simulink model "filt_adapt"  (R2020a)
settings: Solver=VariableStepAuto  StartTime=0.0  StopTime=10.0  RelTol=1e-3
values from neighbouring files (symbols this model uses):
  miu = 0.025    [lab3.m]
  sample_time = 0.03    [lab3.m]
settings Model: Creator=josem  LastModifiedBy=josem

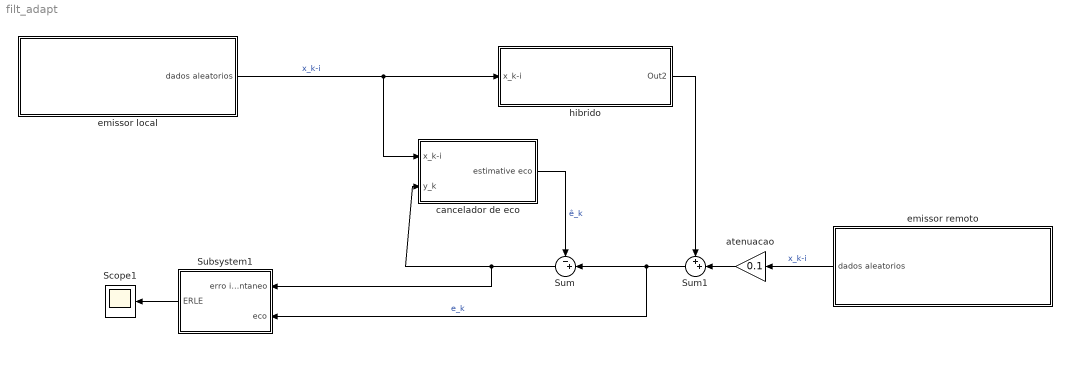
== system filt_adapt ==
  Scope1 : Scope
  Subsystem1 : Subsystem
  Sum : Sum  Inputs=-+|
  Sum1 : Sum  Inputs=++|
  atenuacao : Gain  Gain=0.1
  cancelador de eco : Subsystem
  emissor local : Subsystem
  emissor remoto : Subsystem
  hibrido : Subsystem
  wires:
  emissor local/1(dados aleatorios) -> cancelador de eco/1(x_k-i), hibrido/1(x_k-i)  "x_k-i"
  cancelador de eco/1(estimative eco) -> Sum/1  "ê_k"
  hibrido/1(Out2) -> Sum1/1
  emissor remoto/1(dados aleatorios) -> atenuacao/1  "x_k-i"
  atenuacao/1 -> Sum1/2
  Sum1/1 -> Subsystem1/2(eco), Sum/2  "e_k"
  Subsystem1/1(ERLE) -> Scope1/1
  Sum/1 -> Subsystem1/1(erro instantaneo), cancelador de eco/2(y_k)

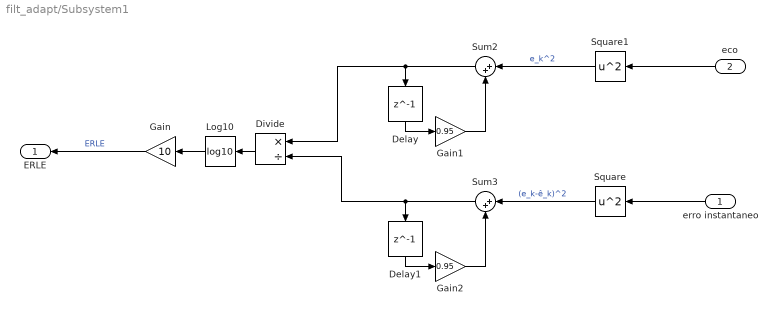
== system filt_adapt/Subsystem1 ==
  erro instantaneo : Inport
  eco : Inport  Port=2
  Delay : Delay  DelayLength=1  InitialCondition=0
  Delay1 : Delay  DelayLength=1  InitialCondition=0
  Divide : Product  Inputs=*/
  Gain : Gain  Gain=10
  Gain1 : Gain  Gain=0.95
  Gain2 : Gain  Gain=0.95
  Log10 : Math  Operator=log10  SaturateOnIntegerOverflow=on
  Square : Math  Operator=square  SaturateOnIntegerOverflow=on
  Square1 : Math  Operator=square  SaturateOnIntegerOverflow=on
  Sum2 : Sum  Inputs=|++
  Sum3 : Sum  Inputs=|++
  ERLE : Outport
  wires:
  Log10/1 -> Gain/1
  erro instantaneo/1 -> Square/1
  Divide/1 -> Log10/1
  eco/1 -> Square1/1
  Square/1 -> Sum3/1  "(e_k-ê_k)^2"
  Gain/1 -> ERLE/1  "ERLE"
  Square1/1 -> Sum2/1  "e_k^2"
  Sum2/1 -> Delay/1, Divide/1
  Delay/1 -> Gain1/1
  Gain1/1 -> Sum2/2
  Gain2/1 -> Sum3/2
  Delay1/1 -> Gain2/1
  Sum3/1 -> Delay1/1, Divide/2

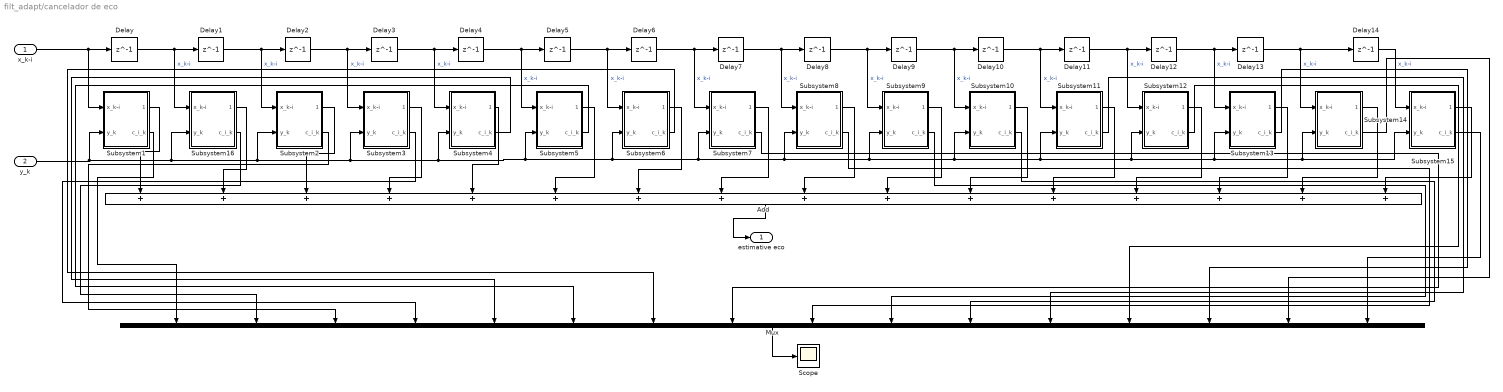
== system filt_adapt/cancelador de eco ==
  x_k-i : Inport
  y_k : Inport  Port=2
  Add : Sum  Inputs=++++++++++++++++
  Delay{,1..14} (15 alike) : Delay  DelayLength=1  InitialCondition=0
  Mux : Mux  Inputs=16
  Scope : Scope
  Subsystem1 : Subsystem
  Subsystem10 : Subsystem
  Subsystem11 : Subsystem
  Subsystem12 : Subsystem
  Subsystem13 : Subsystem
  Subsystem14 : Subsystem
  Subsystem15 : Subsystem
  Subsystem16 : Subsystem
  Subsystem2 : Subsystem
  Subsystem3 : Subsystem
  Subsystem4 : Subsystem
  Subsystem5 : Subsystem
  Subsystem6 : Subsystem
  Subsystem7 : Subsystem
  Subsystem8 : Subsystem
  Subsystem9 : Subsystem
  estimative eco : Outport
  wires:
  Delay8/1 -> Subsystem9/1(x_k-i), Delay9/1  "x_k-i"
  Delay6/1 -> Subsystem7/1(x_k-i), Delay7/1  "x_k-i"
  Delay5/1 -> Subsystem6/1(x_k-i), Delay6/1  "x_k-i"
  Delay12/1 -> Subsystem13/1(x_k-i), Delay13/1  "x_k-i"
  Delay3/1 -> Subsystem4/1(x_k-i), Delay4/1  "x_k-i"
  Delay7/1 -> Subsystem8/1(x_k-i), Delay8/1  "x_k-i"
  Delay1/1 -> Subsystem2/1(x_k-i), Delay2/1  "x_k-i"
  Delay10/1 -> Subsystem11/1(x_k-i), Delay11/1  "x_k-i"
  Delay2/1 -> Subsystem3/1(x_k-i), Delay3/1  "x_k-i"
  Delay/1 -> Subsystem16/1(x_k-i), Delay1/1  "x_k-i"
  Delay4/1 -> Subsystem5/1(x_k-i), Delay5/1  "x_k-i"
  Add/1 -> estimative eco/1
  Delay11/1 -> Subsystem12/1(x_k-i), Delay12/1  "x_k-i"
  Subsystem1/1(x_k-i * c_i_k) -> Add/1
  Subsystem16/1(x_k-i * c_i_k) -> Add/2
  x_k-i/1 -> Subsystem1/1(x_k-i), Delay/1
  Delay9/1 -> Subsystem10/1(x_k-i), Delay10/1  "x_k-i"
  Delay14/1 -> Subsystem15/1(x_k-i)  "x_k-i"
  Delay13/1 -> Subsystem14/1(x_k-i), Delay14/1  "x_k-i"
  y_k/1 -> Subsystem1/2(y_k), Subsystem16/2(y_k), Subsystem2/2(y_k), Subsystem3/2(y_k), Subsystem4/2(y_k), Subsystem5/2(y_k), Subsystem6/2(y_k), Subsystem7/2(y_k), Subsystem8/2(y_k), Subsystem9/2(y_k), Subsystem10/2(y_k), Subsystem11/2(y_k), Subsystem12/2(y_k), Subsystem13/2(y_k), Subsystem15/2(y_k), Subsystem14/2(y_k)
  Subsystem2/1(x_k-i * c_i_k) -> Add/3
  Subsystem3/1(x_k-i * c_i_k) -> Add/4
  Subsystem4/1(x_k-i * c_i_k) -> Add/5
  Subsystem5/1(x_k-i * c_i_k) -> Add/6
  Subsystem6/1(x_k-i * c_i_k) -> Add/7
  Subsystem7/1(x_k-i * c_i_k) -> Add/8
  Subsystem8/1(x_k-i * c_i_k) -> Add/9
  Subsystem9/1(x_k-i * c_i_k) -> Add/10
  Subsystem10/1(x_k-i * c_i_k) -> Add/11
  Subsystem11/1(x_k-i * c_i_k) -> Add/12
  Subsystem12/1(x_k-i * c_i_k) -> Add/13
  Subsystem13/1(x_k-i * c_i_k) -> Add/14
  Subsystem14/1(x_k-i * c_i_k) -> Add/15
  Subsystem15/1(x_k-i * c_i_k) -> Add/16
  Subsystem1/2(c_i_k) -> Mux/1
  Subsystem16/2(c_i_k) -> Mux/2
  Subsystem2/2(c_i_k) -> Mux/3
  Subsystem3/2(c_i_k) -> Mux/4
  Subsystem4/2(c_i_k) -> Mux/5
  Subsystem5/2(c_i_k) -> Mux/6
  Subsystem6/2(c_i_k) -> Mux/7
  Subsystem7/2(c_i_k) -> Mux/8
  Subsystem8/2(c_i_k) -> Mux/9
  Subsystem9/2(c_i_k) -> Mux/10
  Subsystem10/2(c_i_k) -> Mux/11
  Subsystem11/2(c_i_k) -> Mux/12
  Subsystem12/2(c_i_k) -> Mux/13
  Subsystem13/2(c_i_k) -> Mux/14
  Subsystem14/2(c_i_k) -> Mux/15
  Subsystem15/2(c_i_k) -> Mux/16
  Mux/1 -> Scope/1

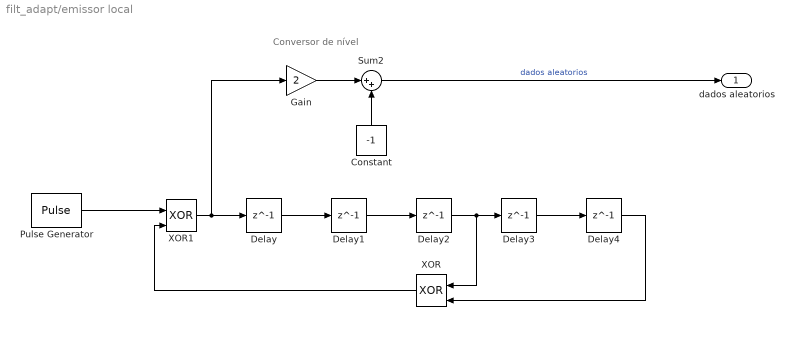
== system filt_adapt/emissor local ==
  note: Conversor de nível
  Constant : Constant  Value=-1
  Delay{,1..4} (5 alike) : Delay  DelayLength=1  InitialCondition=0
  Gain : Gain  Gain=2
  Pulse Generator : DiscretePulseGenerator  SampleTime=sample_time
  Sum2 : Sum  Inputs=|++
  XOR : Logic  Operator=XOR  IconShape=distinctive  AllPortsSameDT=off  OutDataTypeStr=boolean
  XOR1 : Logic  Operator=XOR  IconShape=distinctive  AllPortsSameDT=off  OutDataTypeStr=boolean
  dados aleatorios : Outport
  wires:
  Delay/1 -> Delay1/1
  Delay1/1 -> Delay2/1
  Delay4/1 -> XOR/2
  XOR/1 -> XOR1/2
  Pulse Generator/1 -> XOR1/1
  Delay2/1 -> XOR/1, Delay3/1
  Delay3/1 -> Delay4/1
  Sum2/1 -> dados aleatorios/1  "dados aleatorios"
  Gain/1 -> Sum2/1
  XOR1/1 -> Gain/1, Delay/1
  Constant/1 -> Sum2/2

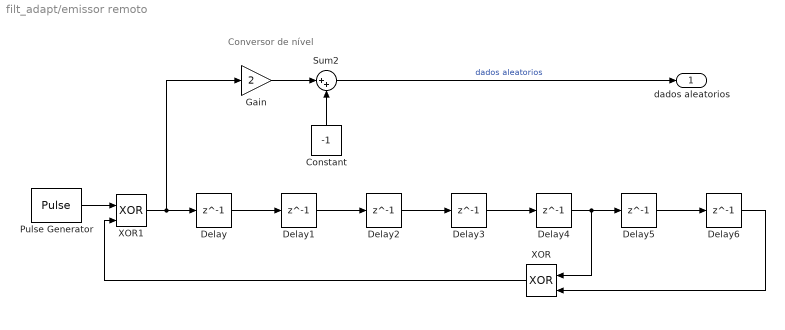
== system filt_adapt/emissor remoto ==
  note: Conversor de nível
  Constant : Constant  Value=-1
  Delay{,1..6} (7 alike) : Delay  DelayLength=1  InitialCondition=0
  Gain : Gain  Gain=2
  Pulse Generator : DiscretePulseGenerator  SampleTime=sample_time
  Sum2 : Sum  Inputs=|++
  XOR : Logic  Operator=XOR  IconShape=distinctive  AllPortsSameDT=off  OutDataTypeStr=boolean
  XOR1 : Logic  Operator=XOR  IconShape=distinctive  AllPortsSameDT=off  OutDataTypeStr=boolean
  dados aleatorios : Outport
  wires:
  Delay/1 -> Delay1/1
  Delay1/1 -> Delay2/1
  XOR/1 -> XOR1/2
  Pulse Generator/1 -> XOR1/1
  Delay2/1 -> Delay3/1
  Constant/1 -> Sum2/2
  XOR1/1 -> Gain/1, Delay/1
  Gain/1 -> Sum2/1
  Sum2/1 -> dados aleatorios/1  "dados aleatorios"
  Delay3/1 -> Delay4/1
  Delay5/1 -> Delay6/1
  Delay4/1 -> XOR/1, Delay5/1
  Delay6/1 -> XOR/2

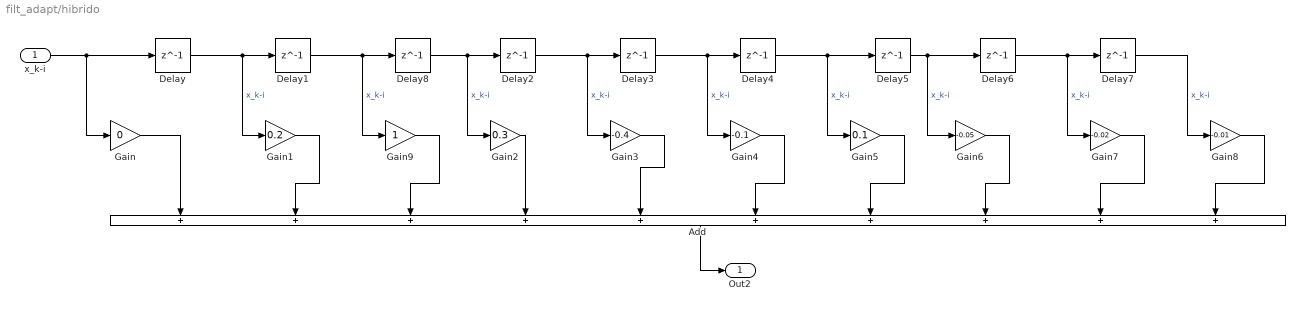
== system filt_adapt/hibrido ==
  x_k-i : Inport
  Add : Sum  Inputs=++++++++++
  Delay{,1..8} (9 alike) : Delay  DelayLength=1  InitialCondition=0
  Gain : Gain  Gain=0
  Gain1 : Gain  Gain=0.2
  Gain2 : Gain  Gain=0.3
  Gain3 : Gain  Gain=-0.4
  Gain4 : Gain  Gain=-0.1
  Gain5 : Gain  Gain=0.1
  Gain6 : Gain  Gain=-0.05
  Gain7 : Gain  Gain=-0.02
  Gain8 : Gain  Gain=-0.01
  Gain9 : Gain
  Out2 : Outport
  wires:
  Delay6/1 -> Gain7/1, Delay7/1  "x_k-i"
  Delay5/1 -> Delay6/1, Gain6/1  "x_k-i"
  Delay3/1 -> Gain4/1, Delay4/1  "x_k-i"
  Delay7/1 -> Gain8/1  "x_k-i"
  Delay8/1 -> Gain2/1, Delay2/1  "x_k-i"
  Delay2/1 -> Gain3/1, Delay3/1  "x_k-i"
  Delay/1 -> Gain1/1, Delay1/1  "x_k-i"
  Delay4/1 -> Gain5/1, Delay5/1  "x_k-i"
  Add/1 -> Out2/1
  x_k-i/1 -> Gain/1, Delay/1
  Delay1/1 -> Gain9/1, Delay8/1  "x_k-i"
  Gain/1 -> Add/1
  Gain1/1 -> Add/2
  Gain9/1 -> Add/3
  Gain2/1 -> Add/4
  Gain3/1 -> Add/5
  Gain4/1 -> Add/6
  Gain5/1 -> Add/7
  Gain6/1 -> Add/8
  Gain7/1 -> Add/9
  Gain8/1 -> Add/10

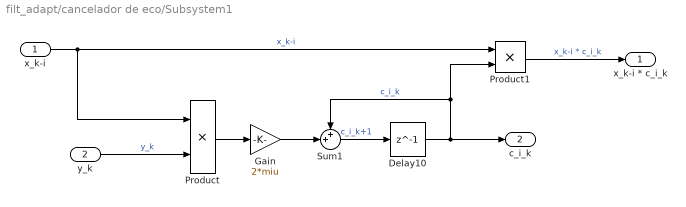
== system filt_adapt/cancelador de eco/Subsystem1 ==
  x_k-i : Inport
  y_k : Inport  Port=2
  Delay10 : Delay  DelayLength=1  InitialCondition=0
  Gain : Gain  Gain=2*miu
  Product : Product
  Product1 : Product
  Sum1 : Sum  Inputs=++|
  x_k-i * c_i_k : Outport
  c_i_k : Outport  Port=2
  wires:
  Product/1 -> Gain/1
  y_k/1 -> Product/2  "y_k"
  Product1/1 -> x_k-i * c_i_k/1  "x_k-i * c_i_k"
  x_k-i/1 -> Product/1, Product1/1  "x_k-i"
  Delay10/1 -> c_i_k/1, Sum1/1, Product1/2  "c_i_k"
  Gain/1 -> Sum1/2
  Sum1/1 -> Delay10/1  "c_i_k+1"

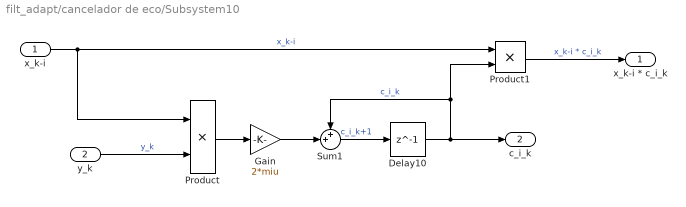
== system filt_adapt/cancelador de eco/Subsystem10 ==
  x_k-i : Inport
  y_k : Inport  Port=2
  Delay10 : Delay  DelayLength=1  InitialCondition=0
  Gain : Gain  Gain=2*miu
  Product : Product
  Product1 : Product
  Sum1 : Sum  Inputs=++|
  x_k-i * c_i_k : Outport
  c_i_k : Outport  Port=2
  wires:
  Product/1 -> Gain/1
  y_k/1 -> Product/2  "y_k"
  Product1/1 -> x_k-i * c_i_k/1  "x_k-i * c_i_k"
  x_k-i/1 -> Product/1, Product1/1  "x_k-i"
  Delay10/1 -> c_i_k/1, Sum1/1, Product1/2  "c_i_k"
  Gain/1 -> Sum1/2
  Sum1/1 -> Delay10/1  "c_i_k+1"

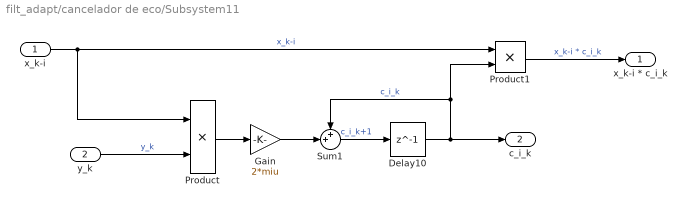
== system filt_adapt/cancelador de eco/Subsystem11 ==
  x_k-i : Inport
  y_k : Inport  Port=2
  Delay10 : Delay  DelayLength=1  InitialCondition=0
  Gain : Gain  Gain=2*miu
  Product : Product
  Product1 : Product
  Sum1 : Sum  Inputs=++|
  x_k-i * c_i_k : Outport
  c_i_k : Outport  Port=2
  wires:
  Product/1 -> Gain/1
  y_k/1 -> Product/2  "y_k"
  Product1/1 -> x_k-i * c_i_k/1  "x_k-i * c_i_k"
  x_k-i/1 -> Product/1, Product1/1  "x_k-i"
  Delay10/1 -> c_i_k/1, Sum1/1, Product1/2  "c_i_k"
  Gain/1 -> Sum1/2
  Sum1/1 -> Delay10/1  "c_i_k+1"

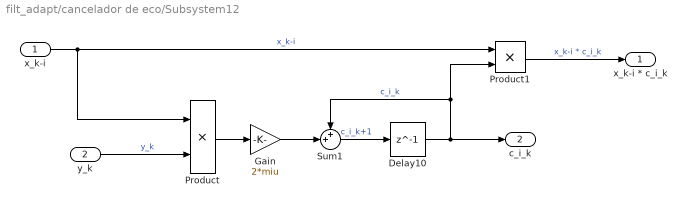
== system filt_adapt/cancelador de eco/Subsystem12 ==
  x_k-i : Inport
  y_k : Inport  Port=2
  Delay10 : Delay  DelayLength=1  InitialCondition=0
  Gain : Gain  Gain=2*miu
  Product : Product
  Product1 : Product
  Sum1 : Sum  Inputs=++|
  x_k-i * c_i_k : Outport
  c_i_k : Outport  Port=2
  wires:
  Product/1 -> Gain/1
  y_k/1 -> Product/2  "y_k"
  Product1/1 -> x_k-i * c_i_k/1  "x_k-i * c_i_k"
  x_k-i/1 -> Product/1, Product1/1  "x_k-i"
  Delay10/1 -> c_i_k/1, Sum1/1, Product1/2  "c_i_k"
  Gain/1 -> Sum1/2
  Sum1/1 -> Delay10/1  "c_i_k+1"

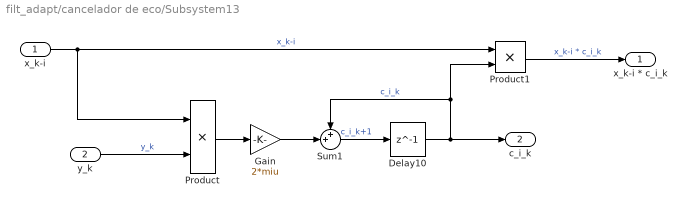
== system filt_adapt/cancelador de eco/Subsystem13 ==
  x_k-i : Inport
  y_k : Inport  Port=2
  Delay10 : Delay  DelayLength=1  InitialCondition=0
  Gain : Gain  Gain=2*miu
  Product : Product
  Product1 : Product
  Sum1 : Sum  Inputs=++|
  x_k-i * c_i_k : Outport
  c_i_k : Outport  Port=2
  wires:
  Product/1 -> Gain/1
  y_k/1 -> Product/2  "y_k"
  Product1/1 -> x_k-i * c_i_k/1  "x_k-i * c_i_k"
  x_k-i/1 -> Product/1, Product1/1  "x_k-i"
  Delay10/1 -> c_i_k/1, Sum1/1, Product1/2  "c_i_k"
  Gain/1 -> Sum1/2
  Sum1/1 -> Delay10/1  "c_i_k+1"

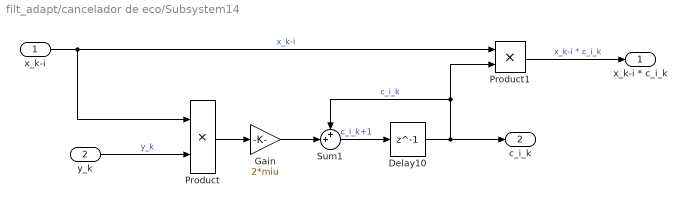
== system filt_adapt/cancelador de eco/Subsystem14 ==
  x_k-i : Inport
  y_k : Inport  Port=2
  Delay10 : Delay  DelayLength=1  InitialCondition=0
  Gain : Gain  Gain=2*miu
  Product : Product
  Product1 : Product
  Sum1 : Sum  Inputs=++|
  x_k-i * c_i_k : Outport
  c_i_k : Outport  Port=2
  wires:
  Product/1 -> Gain/1
  y_k/1 -> Product/2  "y_k"
  Product1/1 -> x_k-i * c_i_k/1  "x_k-i * c_i_k"
  x_k-i/1 -> Product/1, Product1/1  "x_k-i"
  Delay10/1 -> c_i_k/1, Sum1/1, Product1/2  "c_i_k"
  Gain/1 -> Sum1/2
  Sum1/1 -> Delay10/1  "c_i_k+1"

== system filt_adapt/cancelador de eco/Subsystem15 ==
  x_k-i : Inport
  y_k : Inport  Port=2
  Delay10 : Delay  DelayLength=1  InitialCondition=0
  Gain : Gain  Gain=2*miu
  Product : Product
  Product1 : Product
  Sum1 : Sum  Inputs=++|
  x_k-i * c_i_k : Outport
  c_i_k : Outport  Port=2
  wires:
  Product/1 -> Gain/1
  y_k/1 -> Product/2  "y_k"
  Product1/1 -> x_k-i * c_i_k/1  "x_k-i * c_i_k"
  x_k-i/1 -> Product/1, Product1/1  "x_k-i"
  Delay10/1 -> c_i_k/1, Sum1/1, Product1/2  "c_i_k"
  Gain/1 -> Sum1/2
  Sum1/1 -> Delay10/1  "c_i_k+1"

== system filt_adapt/cancelador de eco/Subsystem16 ==
  x_k-i : Inport
  y_k : Inport  Port=2
  Delay10 : Delay  DelayLength=1  InitialCondition=0
  Gain : Gain  Gain=2*miu
  Product : Product
  Product1 : Product
  Sum1 : Sum  Inputs=++|
  x_k-i * c_i_k : Outport
  c_i_k : Outport  Port=2
  wires:
  Product/1 -> Gain/1
  y_k/1 -> Product/2  "y_k"
  Product1/1 -> x_k-i * c_i_k/1  "x_k-i * c_i_k"
  x_k-i/1 -> Product/1, Product1/1  "x_k-i"
  Delay10/1 -> c_i_k/1, Sum1/1, Product1/2  "c_i_k"
  Gain/1 -> Sum1/2
  Sum1/1 -> Delay10/1  "c_i_k+1"

== system filt_adapt/cancelador de eco/Subsystem2 ==
  x_k-i : Inport
  y_k : Inport  Port=2
  Delay10 : Delay  DelayLength=1  InitialCondition=0
  Gain : Gain  Gain=2*miu
  Product : Product
  Product1 : Product
  Sum1 : Sum  Inputs=++|
  x_k-i * c_i_k : Outport
  c_i_k : Outport  Port=2
  wires:
  Product/1 -> Gain/1
  y_k/1 -> Product/2  "y_k"
  Product1/1 -> x_k-i * c_i_k/1  "x_k-i * c_i_k"
  x_k-i/1 -> Product/1, Product1/1  "x_k-i"
  Delay10/1 -> c_i_k/1, Sum1/1, Product1/2  "c_i_k"
  Gain/1 -> Sum1/2
  Sum1/1 -> Delay10/1  "c_i_k+1"

== system filt_adapt/cancelador de eco/Subsystem3 ==
  x_k-i : Inport
  y_k : Inport  Port=2
  Delay10 : Delay  DelayLength=1  InitialCondition=0
  Gain : Gain  Gain=2*miu
  Product : Product
  Product1 : Product
  Sum1 : Sum  Inputs=++|
  x_k-i * c_i_k : Outport
  c_i_k : Outport  Port=2
  wires:
  Product/1 -> Gain/1
  y_k/1 -> Product/2  "y_k"
  Product1/1 -> x_k-i * c_i_k/1  "x_k-i * c_i_k"
  x_k-i/1 -> Product/1, Product1/1  "x_k-i"
  Delay10/1 -> c_i_k/1, Sum1/1, Product1/2  "c_i_k"
  Gain/1 -> Sum1/2
  Sum1/1 -> Delay10/1  "c_i_k+1"

== system filt_adapt/cancelador de eco/Subsystem4 ==
  x_k-i : Inport
  y_k : Inport  Port=2
  Delay10 : Delay  DelayLength=1  InitialCondition=0
  Gain : Gain  Gain=2*miu
  Product : Product
  Product1 : Product
  Sum1 : Sum  Inputs=++|
  x_k-i * c_i_k : Outport
  c_i_k : Outport  Port=2
  wires:
  Product/1 -> Gain/1
  y_k/1 -> Product/2  "y_k"
  Product1/1 -> x_k-i * c_i_k/1  "x_k-i * c_i_k"
  x_k-i/1 -> Product/1, Product1/1  "x_k-i"
  Delay10/1 -> c_i_k/1, Sum1/1, Product1/2  "c_i_k"
  Gain/1 -> Sum1/2
  Sum1/1 -> Delay10/1  "c_i_k+1"

== system filt_adapt/cancelador de eco/Subsystem5 ==
  x_k-i : Inport
  y_k : Inport  Port=2
  Delay10 : Delay  DelayLength=1  InitialCondition=0
  Gain : Gain  Gain=2*miu
  Product : Product
  Product1 : Product
  Sum1 : Sum  Inputs=++|
  x_k-i * c_i_k : Outport
  c_i_k : Outport  Port=2
  wires:
  Product/1 -> Gain/1
  y_k/1 -> Product/2  "y_k"
  Product1/1 -> x_k-i * c_i_k/1  "x_k-i * c_i_k"
  x_k-i/1 -> Product/1, Product1/1  "x_k-i"
  Delay10/1 -> c_i_k/1, Sum1/1, Product1/2  "c_i_k"
  Gain/1 -> Sum1/2
  Sum1/1 -> Delay10/1  "c_i_k+1"

== system filt_adapt/cancelador de eco/Subsystem6 ==
  x_k-i : Inport
  y_k : Inport  Port=2
  Delay10 : Delay  DelayLength=1  InitialCondition=0
  Gain : Gain  Gain=2*miu
  Product : Product
  Product1 : Product
  Sum1 : Sum  Inputs=++|
  x_k-i * c_i_k : Outport
  c_i_k : Outport  Port=2
  wires:
  Product/1 -> Gain/1
  y_k/1 -> Product/2  "y_k"
  Product1/1 -> x_k-i * c_i_k/1  "x_k-i * c_i_k"
  x_k-i/1 -> Product/1, Product1/1  "x_k-i"
  Delay10/1 -> c_i_k/1, Sum1/1, Product1/2  "c_i_k"
  Gain/1 -> Sum1/2
  Sum1/1 -> Delay10/1  "c_i_k+1"

== system filt_adapt/cancelador de eco/Subsystem7 ==
  x_k-i : Inport
  y_k : Inport  Port=2
  Delay10 : Delay  DelayLength=1  InitialCondition=0
  Gain : Gain  Gain=2*miu
  Product : Product
  Product1 : Product
  Sum1 : Sum  Inputs=++|
  x_k-i * c_i_k : Outport
  c_i_k : Outport  Port=2
  wires:
  Product/1 -> Gain/1
  y_k/1 -> Product/2  "y_k"
  Product1/1 -> x_k-i * c_i_k/1  "x_k-i * c_i_k"
  x_k-i/1 -> Product/1, Product1/1  "x_k-i"
  Delay10/1 -> c_i_k/1, Sum1/1, Product1/2  "c_i_k"
  Gain/1 -> Sum1/2
  Sum1/1 -> Delay10/1  "c_i_k+1"

== system filt_adapt/cancelador de eco/Subsystem8 ==
  x_k-i : Inport
  y_k : Inport  Port=2
  Delay10 : Delay  DelayLength=1  InitialCondition=0
  Gain : Gain  Gain=2*miu
  Product : Product
  Product1 : Product
  Sum1 : Sum  Inputs=++|
  x_k-i * c_i_k : Outport
  c_i_k : Outport  Port=2
  wires:
  Product/1 -> Gain/1
  y_k/1 -> Product/2  "y_k"
  Product1/1 -> x_k-i * c_i_k/1  "x_k-i * c_i_k"
  x_k-i/1 -> Product/1, Product1/1  "x_k-i"
  Delay10/1 -> c_i_k/1, Sum1/1, Product1/2  "c_i_k"
  Gain/1 -> Sum1/2
  Sum1/1 -> Delay10/1  "c_i_k+1"

== system filt_adapt/cancelador de eco/Subsystem9 ==
  x_k-i : Inport
  y_k : Inport  Port=2
  Delay10 : Delay  DelayLength=1  InitialCondition=0
  Gain : Gain  Gain=2*miu
  Product : Product
  Product1 : Product
  Sum1 : Sum  Inputs=++|
  x_k-i * c_i_k : Outport
  c_i_k : Outport  Port=2
  wires:
  Product/1 -> Gain/1
  y_k/1 -> Product/2  "y_k"
  Product1/1 -> x_k-i * c_i_k/1  "x_k-i * c_i_k"
  x_k-i/1 -> Product/1, Product1/1  "x_k-i"
  Delay10/1 -> c_i_k/1, Sum1/1, Product1/2  "c_i_k"
  Gain/1 -> Sum1/2
  Sum1/1 -> Delay10/1  "c_i_k+1"
